simulink model "Identification_2degre"  (R2015a)
settings: Solver=ode3  StartTime=0.0  StopTime=10  FixedStep=0.01  RelTol=1e-3
InitFcn:
  | load('LeftOutput_Measures.mat');
  | load('LeftOutput_Measures.mat');
  | Parametres_Rover
undefined symbols (not defined in the file): KL2, TdL2, TwL, ZetaL
settings Model: Creator=tbaroche  LastModifiedBy=tbaroche

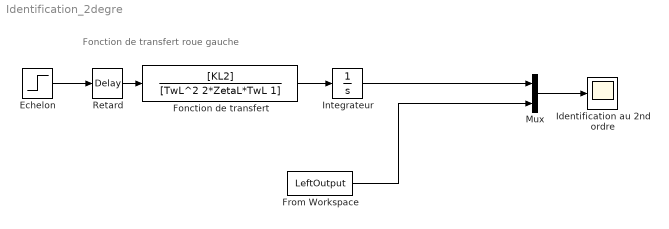
== system Identification_2degre ==
  note: Fonction de transfert roue gauche
  Echelon : Step  Time=3  After=50  SampleTime=0
  Fonction de transfert : TransferFcn  Numerator=[KL2]  Denominator=[TwL^2 2*ZetaL*TwL 1]
  From Workspace : FromWorkspace  VariableName=LeftOutput  SampleTime=0
  Identification au 2nd ordre : Scope
  Integrateur : Integrator
  Mux : Mux  Inputs=2
  Retard : TransportDelay  DelayTime=TdL2
  wires:
  Mux/1 -> Identification au 2nd ordre/1
  Integrateur/1 -> Mux/1
  From Workspace/1 -> Mux/2
  Retard/1 -> Fonction de transfert/1
  Echelon/1 -> Retard/1
  Fonction de transfert/1 -> Integrateur/1
